simulink model "dz"  (R2024a)
settings: Solver=VariableStepAuto  StartTime=0.0  StopTime=550  RelTol=1e-3
libraries: dspfdesign x12, dspmathops x6, dspsnks4 x1, dspvision x1
settings Model: Creator=sebat  LastModifiedBy=sebat

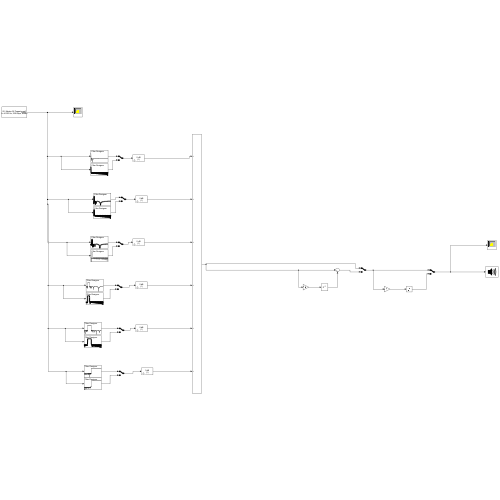
[thumbnail: Simulink's stored preview of the top-level diagram]
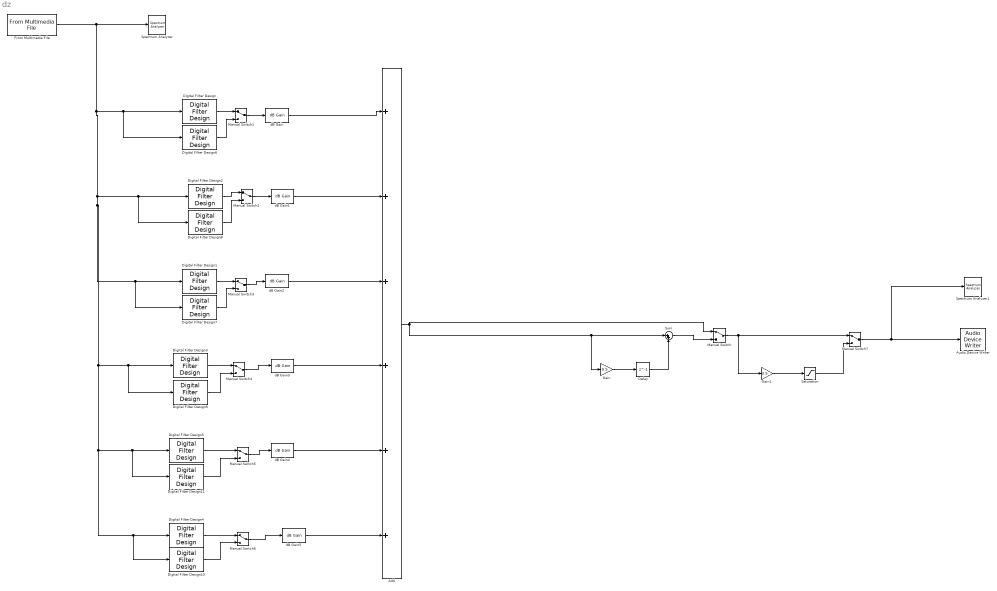
== system dz ==
  Add : Sum  Inputs=++++++
  Audio Device Writer : dspsnks4/Audio Device Writer  Driver=DirectSound  Device=Default  InheritSampleRate=on  SampleRate=44100  BitDepth=16-bit integer  BufferSize=4096  NumBuffers=10  DefaultOutputChannelMapping=on  OutputChannelMapping=1:2  OutputNumUnderrunSamples=off  DriverIdx=1  DeviceWarnFlag=''
  Delay : Delay  DelayLength=1  InitialCondition=0
  Digital Filter Design{,1..11} (12 alike) : dspfdesign/Digital Filter Design  mwdsp_browser_bugfix_var=off
  From Multimedia File : dspvision/From Multimedia File  inputFilename=C:\Users\sebat\OneDrive\Рабочий стол\учеба 5 сем\ЦОС_ДЗ\02. Master Of Puppets.mp3  readRange=[1 Inf]  loop=on  numPlays=inf  outputStreams=Audio only  videoDataType=single  audioDataType=double  inheritSampleTime=on  userDefinedSampleTime=1/30  noAudioOutput=off  isIntensityVideo=off  fourcc=RGB  colorVideoFormat=Separate color signals  outputEOF=off  dataOrg=Column-major  audioFrameSize=1024  computeAudioFrameSize=off  outSamplingMode=Sample based
      settings: LibrarySourceBlock=audiosources/From Multimedia File
  Gain : Gain  Gain=0.5
  Gain1 : Gain  Gain=3.5
  Manual Switch{,1..7} (8 alike) : ManualSwitch
  Saturation : Saturate
  Spectrum Analyzer : SpectrumAnalyzer  WindowPosition=[92.000000,361.000000,800.000000,500.000000,]  ScopeFrameLocation=window  SampleRateSource=Property  SampleRate=44.1e3  PlotAsTwoSidedSpectrum=off  FrequencySpan=Start and stop frequencies  StartFrequency=20  StopFrequency=20e3  YLimits=[-118.35222708,19.08481109]  SelectedToolstripTab=spectrumAnalyzerToolstrip.spectrumTab
  Spectrum Analyzer1 : SpectrumAnalyzer  WindowPosition=[229.000000,776.000000,800.000000,500.000000,]  ScopeFrameLocation=window  SampleRateSource=Property  SampleRate=44.1e3  PlotAsTwoSidedSpectrum=off  FrequencySpan=Start and stop frequencies  StartFrequency=20  StopFrequency=20e3  YLimits=[-110.183412510802,13.563796429197994]  SelectedToolstripTab=spectrumAnalyzerToolstrip.spectrumTab
  Sum : Sum  Inputs=|++
  dB Gain{,1..5} (6 alike) : dspmathops/dB Gain  dB=0  intype=Amplitude
  wires:
  From Multimedia File/1 -> Digital Filter Design10/1, Digital Filter Design4/1, Digital Filter Design11/1, Digital Filter Design5/1, Digital Filter Design9/1, Digital Filter Design3/1, Digital Filter Design7/1, Digital Filter Design1/1, Digital Filter Design8/1, Digital Filter Design2/1, Digital Filter Design6/1, Digital Filter Design/1, Spectrum Analyzer/1
  dB Gain/1 -> Add/1
  dB Gain1/1 -> Add/2
  dB Gain2/1 -> Add/3
  dB Gain3/1 -> Add/4
  Gain/1 -> Delay/1
  Sum/1 -> Manual Switch/2
  Add/1 -> Gain/1, Sum/1, Manual Switch/1
  Delay/1 -> Sum/2
  dB Gain4/1 -> Add/5
  dB Gain5/1 -> Add/6
  Digital Filter Design/1 -> Manual Switch1/1
  Digital Filter Design6/1 -> Manual Switch1/2
  Manual Switch1/1 -> dB Gain/1
  Digital Filter Design2/1 -> Manual Switch2/1
  Digital Filter Design8/1 -> Manual Switch2/2
  Manual Switch2/1 -> dB Gain1/1
  Digital Filter Design7/1 -> Manual Switch3/2
  Digital Filter Design1/1 -> Manual Switch3/1
  Manual Switch3/1 -> dB Gain2/1
  Digital Filter Design9/1 -> Manual Switch4/2
  Digital Filter Design3/1 -> Manual Switch4/1
  Manual Switch4/1 -> dB Gain3/1
  Digital Filter Design5/1 -> Manual Switch5/1
  Digital Filter Design11/1 -> Manual Switch5/2
  Manual Switch5/1 -> dB Gain4/1
  Digital Filter Design4/1 -> Manual Switch6/1
  Digital Filter Design10/1 -> Manual Switch6/2
  Manual Switch6/1 -> dB Gain5/1
  Manual Switch/1 -> Gain1/1, Manual Switch7/1
  Manual Switch7/1 -> Spectrum Analyzer1/1, Audio Device Writer/1
  Gain1/1 -> Saturation/1
  Saturation/1 -> Manual Switch7/2
